simulink model "comunicacionArduinoMatlab"  (R2022a)
settings: Solver=VariableStepAuto  StartTime=0.0  StopTime=200  RelTol=1e-3
undefined symbols (not defined in the file): LF
libraries: instrumentseriallib x3, svdutilitieslib x1
settings Model: Creator=felip  LastModifiedBy=zulet

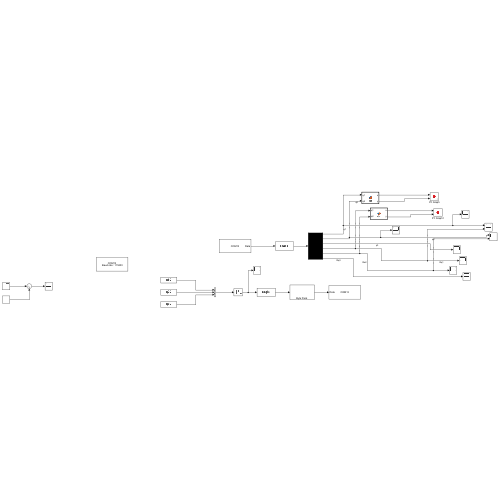
[thumbnail: Simulink's stored preview of the top-level diagram]
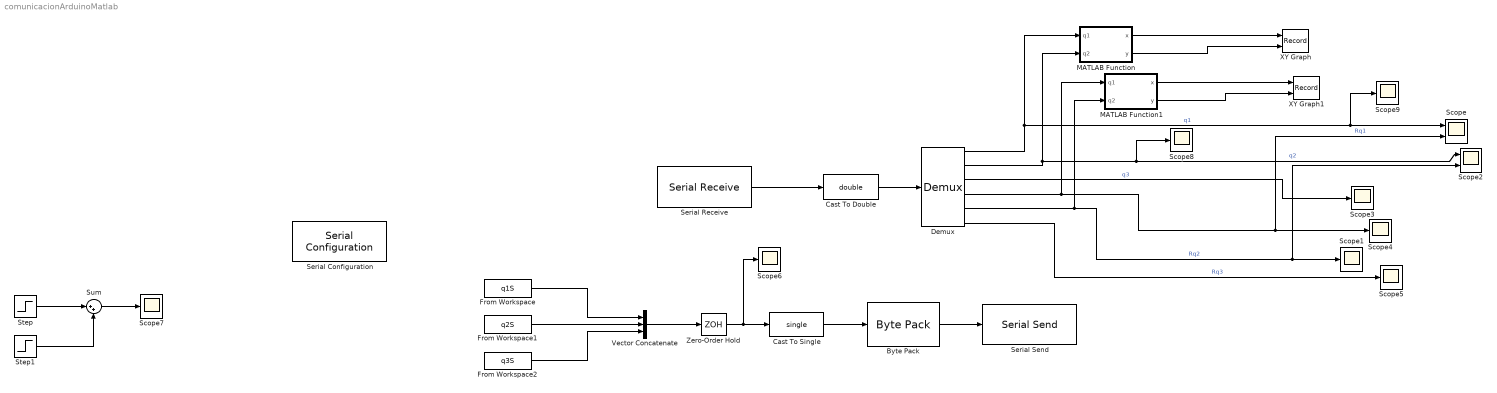
== system comunicacionArduinoMatlab ==
  Byte Pack : svdutilitieslib/Byte Pack  maskPackedDataType=uint32  datatypes={'single'}  byteAlign=4  blockPlatform=arduinoert
      settings: SourceProductBaseCode=ANDROID,ARDUINO,ML_ARDUINO,ECCORTEXA,ECCORTEXR,SC_BEAGLEBONE_BLUE,EC_FREEDOM_BOARD,EC_FRDM_K64F,INTEL_BLOCKSET,MICROBIT,NUCLEO,NVIDIA,PX4AUTOPILOTS,RASPPIIO,STMICRODIS,TIC2000,XILINX_BLOCKSET
  Cast To Double : DataTypeConversion  OutDataTypeStr=double  SaturateOnIntegerOverflow=off  RndMeth=Floor
  Cast To Single : DataTypeConversion  OutDataTypeStr=single  SaturateOnIntegerOverflow=off  RndMeth=Floor
  Demux : Demux  Outputs=6
  From Workspace : FromWorkspace  VariableName=q1S
  From Workspace1 : FromWorkspace  VariableName=q2S
  From Workspace2 : FromWorkspace  VariableName=q3S
  MATLAB Function : MATLAB Function  TreatAsAtomicUnit=on
  MATLAB Function1 : MATLAB Function  TreatAsAtomicUnit=on
  Scope : Scope  NumInputPorts=2
  Scope{1,3..9} (8 alike) : Scope
  Scope2 : Scope  NumInputPorts=2
  Serial Configuration : instrumentseriallib/Serial Configuration  Priority=-200000  PortSel=COM13  Port=COM13  ComPort=COM13  BaudRate=115200  DataBits=8  Parity=none  StopBits=1  ByteOrder=little-endian  FlowControl=none  Timeout=10  SimulateUsing=Interpreted execution  BlockInModel=on  aMode=1
      settings: SourceProductBaseCode=OT,IC,MT
  Serial Receive : instrumentseriallib/Serial Receive  Priority=1  PortSel=COM13  Port=COM13  ComPort=COM13  DataType=single  SaveDataType=uint8  ToggleHeader=on  Header='A'  ToggleTerminator=on  Terminator=LF ('\n')  CustomTerminator=[]  InputFormat=Column major  ToggleDataSize=on  DataSize=[1 6]  EnableBlockingMode=on  ActionDataUnavailable=Output last received value  ActionWhenDataUnavailable=Output last received value  CustomValue=0  SampleTime=0.005  SimulateUsing=Interpreted execution  BlockInModel=on  aMode=1
      settings: SourceProductBaseCode=OT,IC,MT
  Serial Send : instrumentseriallib/Serial Send  Priority=1  PortSel=COM13  Port=COM13  ComPort=COM13  Header='R'  Terminator=LF ('\n')  CustomTerminator=[]  EnableBlockingMode=on  SimulateUsing=Interpreted execution  BlockInModel=on  aMode=1
      settings: SourceProductBaseCode=OT,IC,MT
  Step : Step  Time=0  After=165  SampleTime=0
  Step1 : Step  Time=5  After=-15  SampleTime=0
  Sum : Sum  Inputs=|++
  Vector Concatenate : Concatenate  NumInputs=3
  XY Graph : Record  FileSettingsInternal="{\"entries\":[{\"content\":{\"excelSettings\":{\"content\":{},\"type\":\"Streamout.ExcelSettings\"}},\"type\":\"Streamout.FileSettingStorage\",\"uuid\":\"20c14fec-55a1-446c-a4d6-0391842884f2\"}],\"packageUris\":[\"http://schema.mathworks.com/mf0/streamout_blocks/R2020a\"],\"version\":\"1.0\"}"  Layout=[1 1]  SignalsInternal="{\"entries\":[{\"content\":{\"signals\":[{\"content\":{\"blockPath\":[\"comunicacionArduinoMatlab/XY Graph\"],\"channel\":[],\"dimensions\":[1],\"domain\":\"comunicacionArduinoMatlab/XY Graph\",\"lineColor\":\"#77ac30\",\"plots\":[],\"port\":1,\"sid\":[\"\"],\"signalID\":45,\"signalName\":\"MATLAB Function:1\"},\"type\":\"RecordBlkView.Signal\",\"uuid\":\"6175d4ea-c254-43ab-84d8-b0406e82bca8\"},{\"content\":{\"blockPath\":[\"comunicacionArduinoMatlab/XY Graph\"],\"channel\":[],\"dimensions\":[1],\"domain\":\"comunicacionArduinoMatlab/XY Graph\",\"lineColor\":\"#4dbeee\",\"plots\":[],\"port\":2,\"sid\":[\"\"],\"signalID\":49,\"signalName\":\"MATLAB Function:2\"},\"type\":\"RecordBlkView.Signal\",\"uuid\":\"3c44f669-4397-4260-81ef-269bc63aeb8a\"}]},\"type\":\"RecordBlkView.InputSignals\",\"uuid\":\"68d70c7a-6c3d-4c23-a24f-666559649f94\"}],\"packageUris\":[\"http://schema.mathworks.com/mf0/streamout_blocks/R2020a\"],\"version\":\"1.0\"}"  VisualizationBindings="{\"xyplotplugin\":{\"info\":[{\"series\":[],\"subplotID\":1}]}}"  CompatibilityTag=XY
  XY Graph1 : Record  FileSettingsInternal="{\"entries\":[{\"content\":{\"excelSettings\":{\"content\":{},\"type\":\"Streamout.ExcelSettings\"}},\"type\":\"Streamout.FileSettingStorage\",\"uuid\":\"d06d7c65-01e4-499e-af87-b0d8700c8e8d\"}],\"packageUris\":[\"http://schema.mathworks.com/mf0/streamout_blocks/R2020a\"],\"version\":\"1.0\"}"  Layout=[1 1]  SignalsInternal="{\"entries\":[{\"content\":{\"signals\":[{\"content\":{\"blockPath\":[\"comunicacionArduinoMatlab/XY Graph1\"],\"channel\":[],\"dimensions\":[1],\"domain\":\"comunicacionArduinoMatlab/XY Graph1\",\"lineColor\":\"#a2142f\",\"plots\":[],\"port\":1,\"sid\":[\"\"],\"signalID\":53,\"signalName\":\"MATLAB Function1:1\"},\"type\":\"RecordBlkView.Signal\",\"uuid\":\"bf3ae6e4-cfc9-4b36-af2d-d20a12da71ac\"},{\"content\":{\"blockPath\":[\"comunicacionArduinoMatlab/XY Graph1\"],\"channel\":[],\"dimensions\":[1],\"domain\":\"comunicacionArduinoMatlab/XY Graph1\",\"lineColor\":\"#139fff\",\"plots\":[],\"port\":2,\"sid\":[\"\"],\"signalID\":57,\"signalName\":\"MATLAB Function1:2\"},\"type\":\"RecordBlkView.Signal\",\"uuid\":\"62d4f8bc-60ce-4108-a0db-2f5232357278\"}]},\"type\":\"RecordBlkView.InputSignals\",\"uuid\":\"3bbe185d-c539-437c-9286-a5a70d5d063f\"}],\"packageUris\":[\"http://schema.mathworks.com/mf0/streamout_blocks/R2020a\"],\"version\":\"1.0\"}"  VisualizationBindings="{\"xyplotplugin\":{\"info\":[{\"series\":[],\"subplotID\":1}]}}"  CompatibilityTag=XY
  Zero-Order Hold : ZeroOrderHold  SampleTime=0.005
  wires:
  Serial Receive/1 -> Cast To Double/1
  Zero-Order Hold/1 -> Scope6/1, Cast To Single/1
  Cast To Single/1 -> Byte Pack/1
  Byte Pack/1 -> Serial Send/1
  Vector Concatenate/1 -> Zero-Order Hold/1
  Demux/1 -> MATLAB Function/1(q1), Scope9/1, Scope/1  "q1"
  Demux/5 -> MATLAB Function1/2(q2), Scope2/2, Scope1/1  "Rq2"
  Demux/2 -> MATLAB Function/2(q2), Scope8/1, Scope2/1  "q2"
  From Workspace1/1 -> Vector Concatenate/2
  From Workspace2/1 -> Vector Concatenate/3
  Demux/3 -> Scope3/1  "q3"
  Demux/4 -> MATLAB Function1/1(q1), Scope/2, Scope4/1  "Rq1"
  Demux/6 -> Scope5/1  "Rq3"
  Cast To Double/1 -> Demux/1
  Step/1 -> Sum/1
  Step1/1 -> Sum/2
  Sum/1 -> Scope7/1
  MATLAB Function/1(x) -> XY Graph/1
  MATLAB Function/2(y) -> XY Graph/2
  MATLAB Function1/1(x) -> XY Graph1/1
  MATLAB Function1/2(y) -> XY Graph1/2
  From Workspace/1 -> Vector Concatenate/1

== matlab function comunicacionArduinoMatlab/MATLAB Function ==
  data: x output; q1 input; y output; q2 input
function [x,y] = fcn(q1,q2)
l1=18;
l2=19;
x=l1*cosd(q1)+l2*cosd(q1+q2);
y=l1*sind(q1)+l2*sind(q1+q2);

== matlab function comunicacionArduinoMatlab/MATLAB Function1 ==
  data: x output; q1 input; y output; q2 input
function [x,y] = fcn(q1,q2)
l1=18;
l2=19;
x=l1*cosd(q1)+l2*cosd(q1+q2);
y=l1*sind(q1)+l2*sind(q1+q2);
